simulink model "pendulum_model"  (R2019a)
settings: Solver=VariableStepAuto  StartTime=0.0  StopTime=1000  MaxStep=0.01  RelTol=1e-3
undefined symbols (not defined in the file or in its folder): c, v
settings Model: Creator=Rike Voltz  LastModifiedBy=Rike Voltz

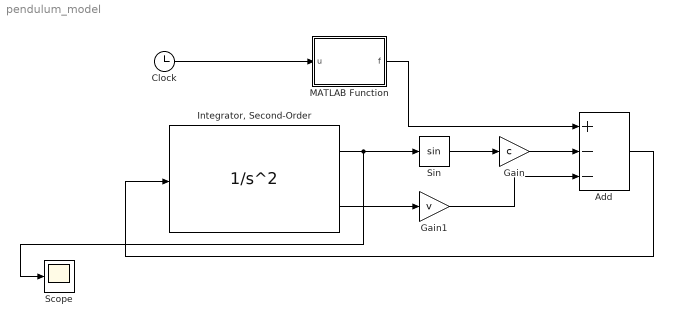
== system pendulum_model ==
  Add : Sum  Inputs=+--
  Clock : Clock
  Gain : Gain  Gain=c
  Gain1 : Gain  Gain=v
  "Integrator, Second-Order" : SecondOrderIntegrator  ICX=0.01
  MATLAB Function : MATLAB Function  TreatAsAtomicUnit=on
  Scope : Scope
  Sin : Trigonometry
  wires:
  Sin/1 -> Gain/1
  "Integrator, Second-Order"/2 -> Gain1/1
  Gain1/1 -> Add/3
  Gain/1 -> Add/2
  Add/1 -> "Integrator, Second-Order"/1
  MATLAB Function/1(f) -> Add/1
  Clock/1 -> MATLAB Function/1(u)
  "Integrator, Second-Order"/1 -> Scope/1, Sin/1

== matlab function pendulum_model/MATLAB Function ==
  data: u input; f output
function f = fcn(u)
f=sin(u);
end
